simulink model "Case3_IEEE39_UGFLandGFM"  (R2024a)
settings: Solver=VariableStepAuto  StartTime=0.0  StopTime=30  RelTol=1e-3
InitFcn:
  | IEEE39data_UGFLandGFM;
values from neighbouring files (symbols this model uses):
  Fref = 60    [IEEE39data_UGFLandGFM.m]
  IBR = [ ... (first row only)    [IEEE39data_UGFLandGFM.m]
  line = [     1	2	0.0035	0.0411	0.6987	0	1	22 ... (first row only)    [IEEE39data_UGFLandGFM.m]
  Sbase = 1e6    (= 1000000)    [IEEE39data_UGFLandGFM.m]
  SG = [ ... (first row only)    [IEEE39data_UGFLandGFM.m]
  UGFML = [ ... (first row only)    [IEEE39data_UGFLandGFM.m]
  Vbase = 22e3    (= 22000)    [IEEE39data_UGFLandGFM.m]
libraries: spsThreePhaseVIMeasurementLib x66, spsThreePhasePISectionLineLib x35, spsPLL3phLib x25, spsControlledVoltageSourceLib x21, spsThreePhaseParallelRLCLoadLib x21, powerlib_extras x20, spsGroundLib x20, spsMeanLib x20, spsRMSLib x15, spsabctodq0Lib x11, spsThreePhaseSeriesRLCBranchLib x10, slpidlib x10
(part 2 of 5)

== system Case3_IEEE39_UGFLandGFM/SG1 ==
  3-phase Instantaneous Active & Reactive Power4 : powerlib_extras/Measurements/3-phase  Instantaneous  Active & Reactive Power
  Add : Sum  Inputs=+-
  Add1 : Sum  Inputs=-+
  Constant1 : Constant  Value=SG(1,6)
  Constant2 : Constant  Value=Fref
  Constant3 : Constant  Value=SG(1,4)
  Constant6 : Constant  Value=SG(1,7)
  Demux : Demux  Outputs=2
  Demux1 : Demux  Outputs=2
  Divide : Product  Inputs=*/
  Gain1 : Gain  Gain=0.2
  Gain2 : Gain  Gain=1.732/22000
  Mean : spsMeanLib/Mean  Freq=60  Vinit=0  Ts=1e-4
  PID Controller1 : slpidlib/PID Controller  Controller=PI  Form=Parallel  TimeDomain=Discrete-time  UseExternalTs=off  SampleTime=5e-4  IntegratorMethod=Forward Euler  FilterMethod=Forward Euler  ControllerParametersSource=internal  P=5  I=30  UseKiTs=off  D=0  UseExternalDerivativeSource=off  N=100  UseFilter=on  TunerSelectOption=Transfer Function Based (PID Tuner App)  InitialConditionSource=internal  InitialConditionForIntegrator=1  InitialConditionForFilter=0  DifferentiatorICPrevScaledInput=0  ExternalReset=level  TrackingMode=off  Kt=1  LimitOutput=off  SatLimitsSource=internal  UpperSaturationLimit=inf  LowerSaturationLimit=-inf  LinearizeAsGain=on  AntiWindupMode=none  Kb=1  LimitIntegrator=off  UpperIntegratorSaturationLimit=inf  LowerIntegratorSaturationLimit=-inf  POutMin=[]  POutMax=[]  IOutMin=[]  IOutMax=[]  DOutMin=[]  DOutMax=[]  NOutMin=[]  NOutMax=[]  SumOutMin=[]  SumOutMax=[]  SaturationOutMin=[]  SaturationOutMax=[]  PParamMin=[]  PParamMax=[]  IParamMin=[]  IParamMax=[]  DParamMin=[]  DParamMax=[]  NParamMin=[]  NParamMax=[]  KbParamMin=[]  KbParamMax=[]  KtParamMin=[]  KtParamMax=[]  KbOutMin=[]  KbOutMax=[]  KtOutMin=[]  KtOutMax=[]  IntegratorOutMin=[]  IntegratorOutMax=[]  FilterOutMin=[]  FilterOutMax=[]  SumI1OutMin=[]  SumI1OutMax=[]  SumI2OutMin=[]  SumI2OutMax=[]  SumI3OutMin=[]  SumI3OutMax=[]  SumI4OutMin=[]  SumI4OutMax=[]  SumDOutMin=[]  SumDOutMax=[]  DifferentiatorOutMin=[]  DifferentiatorOutMax=[]  FilterDiffOutCoefMin=[]  FilterDiffOutCoefMax=[]  ReciprocalOutMin=[]  ReciprocalOutMax=[]  SumDenOutMin=[]  SumDenOutMax=[]  SumNumOutMin=[]  SumNumOutMax=[]  DivideOutMin=[]  DivideOutMax=[]  UdiffTsProdOutMin=[]  UdiffTsProdOutMax=[]  NTsProdOutMin=[]  NTsProdOutMax=[]  UintegralTsProdOutMin=[]  UintegralTsProdOutMax=[]  UngainTsProdOutMin=[]  UngainTsProdOutMax=[]  ClampingZeroOutDataTypeStr=Inherit: Inherit via back propagation  ClampingZeroOutMin=[]  ClampingZeroOutMax=[]  FilterDenConstantOutDataTypeStr=Inherit: Inherit via back propagation  FilterDenConstantOutMin=[]  FilterDenConstantOutMax=[]  PCopyOutDataTypeStr=Inherit: Inherit via back propagation  PCopyOutMin=[]  PCopyOutMax=[]  NCopyOutDataTypeStr=Inherit: Inherit via back propagation  NCopyOutMin=[]  NCopyOutMax=[]  IntegratorContinuousStateAttributes=''  IntegratorStateMustResolveToSignalObject=off  IntegratorRTWStateStorageClass=Auto  FilterContinuousStateAttributes=''  FilterStateMustResolveToSignalObject=off  FilterRTWStateStorageClass=Auto  ParallelPVariant=InternalParameters  IdealPVariant=Disabled  IVariant=InternalParameters  DVariant=Disabled  IntegratorVariant=Discrete  SatVariant=Disabled  AWVariant=Passthrough  PCopyVariant=Disabled  TRVariant=Disabled  FdbkBlocksVariant=Forward  IdealPFdbkVariant=Disabled  SatFdbkVariant=Disabled  DerivativeFilterVariant=Disabled  NVariant=Disabled  NCopyVariant=Disabled_SignalSpec  FilterICVariant=Disabled  IntegratorICVariant=InternalICs  ExternalResetVariant=ExternalReset  TRSumVariant=Passthrough  SumFdbkVariant=Disabled  SumVariant=Sum_PI  TsampFilterVariant=InternalTs  TsampNgainVariant=Passthrough  TsampIntegralVariant=Disabled_SignalSpec  ExternalSaturationOutDataTypeStr=Inherit: Same as second input  DerivativeSourceVariant=Disabled
  PLL (3ph) : spsPLL3phLib/PLL (3ph)  Fmin=59.5  Par_Init=[0, 60]  ParK=[180, 3200, 1]  TcD=1e-4  MaxRateChangeFreq=12  FilterCutOffFreq=25  Ts=1e-5  AGC=on
  Product : Product
  RMS Measurement : eeRmsMeasurement/RMS Measurement  LabelModeActiveChoice=Total  F=60  SpecifyHarmonics=off  K=[0 1 2]  Ts=1e-4
      settings: LibrarySourceBlock=|
      | ee_sl_lib/Measurements/RMS
      | Measurement
  Saturation : Saturate  UpperLimit=1.2  LowerLimit=0.1
  Saturation2 : Saturate  UpperLimit=5  LowerLimit=0.5
  Scope : Scope  NumInputPorts=5
  Scope1 : Scope
  Step : Step  Before=1  After=0  SampleTime=0
  Sum : Sum  Inputs=|+-
  Synchronous Machine pu Standard : spsSynchronousMachinepuStandardLib/Synchronous Machine pu Standard  PresetModel=No  MechanicalLoad=Mechanical power Pm  ShowDetailedParameters=on  RotorType=Salient-pole  Units=per unit standard parameters  MeasurementBus=off  NominalParameters=[5e6 22000 60]  Reactances1=[ 1.81, 0.3, 0.23, 1.76, 0.65, 0.25, 0.15 ]  Reactances2=[2.24 0.17 0.12 1.02 0.13 0.08]  dAxisTimeConstants=Short-circuit  qAxisTimeConstants=Short-circuit  TimeConstants1="[ 4.4849  0.0681  0.1  ]"  TimeConstants2=[ 8.0, 0.03, 1.0, 0.07 ]  TimeConstants3="[  4.49  0.0681  0.0513  ]"  TimeConstants4=[ 8.0, 0.03, 0.3371, 0.0295 ]  TimeConstants5=[ 1.01, 0.053, 0.1 ]  TimeConstants6=[ 1.3201, 0.023, 1.0, 0.07 ]  TimeConstants7=[0.012 0.003 0.003]  TimeConstants8=[ 1.3201, 0.0231, 0.3371, 0.0295 ]  StatorResistance=0.037875  Mechanical=[SG(1,5) 0.02056 2]  PolePairs=20  InitialConditions="[ 0  0  0  0  0  0  0  0  1 ]"  SetSaturation=on  Saturation=[0.6404,0.7127,0.8441,0.9214,0.9956,1.082,1.19,1.316,1.457;0.7,0.7698,0.8872,0.9466,0.9969,1.046,1.1,1.151,1.201]  LoadFlowParameters=[1,0,0,0,0]  TsPowergui=0  TsBlock=-1  IterativeModel=Trapezoidal non iterative  IterativeDiscreteModel=Trapezoidal non iterative  BusType=PV  Pref=0  Qref=0  Qmin=-inf  Qmax=inf  PLF=0  QLF=0
  Three-Phase V-I Measurement3 : spsThreePhaseVIMeasurementLib/Three-Phase V-I Measurement  VoltageMeasurement=phase-to-ground  SetLabelV=off  LabelV=Vabc  Vpu=off  VpuLL=off  CurrentMeasurement=yes  SetLabelI=off  LabelI=Iabc  Ipu=off  Pbase=1e5  Vbase=380  OutputType=Complex  PhasorSimulation=off  PSBequivalent=0
  Transfer Fcn : TransferFcn  Denominator=[0.6 1]
  Conn1 : PMIOPort  Side=Right
  Conn2 : PMIOPort  Port=2  Side=Right
  Conn3 : PMIOPort  Port=3  Side=Right
  tag scope: P_Bus30=global, Q_Bus30=global, V_Bus30=global
  wires:
  3-phase Instantaneous Active & Reactive Power4/1 -> Mean/1
  Three-Phase V-I Measurement3/1 -> 3-phase Instantaneous Active & Reactive Power4/1, RMS Measurement/1, PLL (3ph)/1, Scope/1
  Three-Phase V-I Measurement3/2 -> Scope/2, 3-phase Instantaneous Active & Reactive Power4/2
  Mean/1 -> Demux1/1, Scope/3
  Add1/1 -> Gain1/1
  [SG_Freq] -> Add/1
  Constant2/1 -> Divide/2, Add/2
  Add/1 -> Divide/1
  Divide/1 -> Transfer Fcn/1
  Constant3/1 -> Product/2
  Constant1/1 -> Add1/2
  Product/1 -> Add1/1
  Transfer Fcn/1 -> Product/1
  Gain1/1 -> Saturation/1
  Gain2/1 -> Demux/1, Scope/4
  RMS Measurement/1 -> Gain2/1
  Demux/1 -> [V_Bus30], [VSG_pu]
  Constant6/1 -> Sum/1
  [VSG_pu] -> Sum/2
  PID Controller1/1 -> Saturation2/1
  Sum/1 -> PID Controller1/1
  Saturation/1 -> Synchronous Machine pu Standard/1
  PLL (3ph)/1 -> Scope/5, [SG_Freq]
  Demux1/1 -> [P_Bus30]
  Demux1/2 -> [Q_Bus30]
  Saturation2/1 -> Synchronous Machine pu Standard/2, Scope1/1
  Step/1 -> PID Controller1/2
  connections:
  Three-Phase V-I Measurement3/RConn1 -- Conn1/RConn1
  Three-Phase V-I Measurement3/RConn2 -- Conn2/RConn1
  Three-Phase V-I Measurement3/RConn3 -- Conn3/RConn1
  Three-Phase V-I Measurement3/LConn1 -- Synchronous Machine pu Standard/RConn1
  Three-Phase V-I Measurement3/LConn2 -- Synchronous Machine pu Standard/RConn2
  Three-Phase V-I Measurement3/LConn3 -- Synchronous Machine pu Standard/RConn3

== system Case3_IEEE39_UGFLandGFM/SG2 ==
  3-phase Instantaneous Active & Reactive Power4 : powerlib_extras/Measurements/3-phase  Instantaneous  Active & Reactive Power
  Add : Sum  Inputs=+-
  Add1 : Sum  Inputs=-+
  Constant1 : Constant  Value=SG(2,6)
  Constant2 : Constant  Value=Fref
  Constant3 : Constant  Value=SG(2,4)
  Constant5 : Constant  Commented=on  Value=1.1
  Constant6 : Constant  Value=SG(2,7)
  DC1A Excitation System : spsDC1AExcitationSystemLib/DC1A Excitation System  Commented=on  Tr=20e-3  KaTa=[460 0.006]  VRminmax=[-0.9 1.0]  KfTf=[0.05 1.5]  TbTc=[0 0]  KeTe=[0.05 0.46]  Efd12=[3.1 2.3]  SeEfd12=[0.33 0.10]  v0=[1 1.8]  TsBlock=0
      settings: LibrarySourceBlock=|
      | sps_lib/Electrical Machines/Synchronous Machine Control/DC1A
      | Excitation System
  Demux : Demux  Outputs=3
  Demux1 : Demux  Outputs=2
  Divide : Product  Inputs=*/
  From1 : From  Commented=on  GotoTag=VSG_pu
  Gain1 : Gain  Gain=0.2
  Gain2 : Gain  Gain=sqrt(3)/22000
  Ground : Ground  Commented=on
  Mean : spsMeanLib/Mean  Freq=60  Vinit=0  Ts=1e-4
  PID Controller1 : slpidlib/PID Controller  Controller=PI  Form=Parallel  TimeDomain=Discrete-time  UseExternalTs=off  SampleTime=5e-4  IntegratorMethod=Forward Euler  FilterMethod=Forward Euler  ControllerParametersSource=internal  P=5  I=30  UseKiTs=off  D=0  UseExternalDerivativeSource=off  N=100  UseFilter=on  TunerSelectOption=Transfer Function Based (PID Tuner App)  InitialConditionSource=internal  InitialConditionForIntegrator=1.8  InitialConditionForFilter=0  DifferentiatorICPrevScaledInput=0  ExternalReset=none  TrackingMode=off  Kt=1  LimitOutput=off  SatLimitsSource=internal  UpperSaturationLimit=inf  LowerSaturationLimit=-inf  LinearizeAsGain=on  AntiWindupMode=none  Kb=1  LimitIntegrator=off  UpperIntegratorSaturationLimit=inf  LowerIntegratorSaturationLimit=-inf  POutMin=[]  POutMax=[]  IOutMin=[]  IOutMax=[]  DOutMin=[]  DOutMax=[]  NOutMin=[]  NOutMax=[]  SumOutMin=[]  SumOutMax=[]  SaturationOutMin=[]  SaturationOutMax=[]  PParamMin=[]  PParamMax=[]  IParamMin=[]  IParamMax=[]  DParamMin=[]  DParamMax=[]  NParamMin=[]  NParamMax=[]  KbParamMin=[]  KbParamMax=[]  KtParamMin=[]  KtParamMax=[]  KbOutMin=[]  KbOutMax=[]  KtOutMin=[]  KtOutMax=[]  IntegratorOutMin=[]  IntegratorOutMax=[]  FilterOutMin=[]  FilterOutMax=[]  SumI1OutMin=[]  SumI1OutMax=[]  SumI2OutMin=[]  SumI2OutMax=[]  SumI3OutMin=[]  SumI3OutMax=[]  SumI4OutMin=[]  SumI4OutMax=[]  SumDOutMin=[]  SumDOutMax=[]  DifferentiatorOutMin=[]  DifferentiatorOutMax=[]  FilterDiffOutCoefMin=[]  FilterDiffOutCoefMax=[]  ReciprocalOutMin=[]  ReciprocalOutMax=[]  SumDenOutMin=[]  SumDenOutMax=[]  SumNumOutMin=[]  SumNumOutMax=[]  DivideOutMin=[]  DivideOutMax=[]  UdiffTsProdOutMin=[]  UdiffTsProdOutMax=[]  NTsProdOutMin=[]  NTsProdOutMax=[]  UintegralTsProdOutMin=[]  UintegralTsProdOutMax=[]  UngainTsProdOutMin=[]  UngainTsProdOutMax=[]  ClampingZeroOutDataTypeStr=Inherit: Inherit via back propagation  ClampingZeroOutMin=[]  ClampingZeroOutMax=[]  FilterDenConstantOutDataTypeStr=Inherit: Inherit via back propagation  FilterDenConstantOutMin=[]  FilterDenConstantOutMax=[]  PCopyOutDataTypeStr=Inherit: Inherit via back propagation  PCopyOutMin=[]  PCopyOutMax=[]  NCopyOutDataTypeStr=Inherit: Inherit via back propagation  NCopyOutMin=[]  NCopyOutMax=[]  IntegratorContinuousStateAttributes=''  IntegratorStateMustResolveToSignalObject=off  IntegratorRTWStateStorageClass=Auto  FilterContinuousStateAttributes=''  FilterStateMustResolveToSignalObject=off  FilterRTWStateStorageClass=Auto  ParallelPVariant=InternalParameters  IdealPVariant=Disabled  IVariant=InternalParameters  DVariant=Disabled  IntegratorVariant=Discrete  SatVariant=Disabled  AWVariant=Passthrough  PCopyVariant=Disabled  TRVariant=Disabled  FdbkBlocksVariant=Forward  IdealPFdbkVariant=Disabled  SatFdbkVariant=Disabled  DerivativeFilterVariant=Disabled  NVariant=Disabled  NCopyVariant=Disabled_SignalSpec  FilterICVariant=Disabled  IntegratorICVariant=InternalICs  ExternalResetVariant=Disabled  TRSumVariant=Passthrough  SumFdbkVariant=Disabled  SumVariant=Sum_PI  TsampFilterVariant=InternalTs  TsampNgainVariant=Passthrough  TsampIntegralVariant=Disabled_SignalSpec  ExternalSaturationOutDataTypeStr=Inherit: Same as second input  DerivativeSourceVariant=Disabled
  PLL (3ph) : spsPLL3phLib/PLL (3ph)  Fmin=59.5  Par_Init=[0, 60]  ParK=[180, 3200, 1]  TcD=1e-4  MaxRateChangeFreq=12  FilterCutOffFreq=25  Ts=1e-5  AGC=on
  Product : Product
  RMS Measurement : eeRmsMeasurement/RMS Measurement  LabelModeActiveChoice=Total  F=60  SpecifyHarmonics=off  K=[0 1 2]  Ts=1e-4
      settings: LibrarySourceBlock=|
      | ee_sl_lib/Measurements/RMS
      | Measurement
  Saturation : Saturate  UpperLimit=0.9  LowerLimit=0.1
  Saturation1 : Saturate  Commented=on  UpperLimit=4  LowerLimit=1.5
  Saturation2 : Saturate  UpperLimit=5  LowerLimit=0.9
  Scope : Scope  NumInputPorts=5
  Scope{1..4} (4 alike) : Scope
  Sum : Sum  Inputs=|+-
  Synchronous Machine pu Standard : spsSynchronousMachinepuStandardLib/Synchronous Machine pu Standard  PresetModel=No  MechanicalLoad=Mechanical power Pm  ShowDetailedParameters=on  RotorType=Salient-pole  Units=per unit standard parameters  MeasurementBus=off  NominalParameters=[5e6 22000 60]  Reactances1=[ 1.81, 0.3, 0.23, 1.76, 0.65, 0.25, 0.15 ]  Reactances2=[2.24 0.17 0.12 1.02 0.13 0.08]  dAxisTimeConstants=Short-circuit  qAxisTimeConstants=Short-circuit  TimeConstants1="[ 4.4849  0.0681  0.1  ]"  TimeConstants2=[ 8.0, 0.03, 1.0, 0.07 ]  TimeConstants3="[  4.49  0.0681  0.0513  ]"  TimeConstants4=[ 8.0, 0.03, 0.3371, 0.0295 ]  TimeConstants5=[ 1.01, 0.053, 0.1 ]  TimeConstants6=[ 1.3201, 0.023, 1.0, 0.07 ]  TimeConstants7=[0.012 0.003 0.003]  TimeConstants8=[ 1.3201, 0.0231, 0.3371, 0.0295 ]  StatorResistance=0.037875  Mechanical=[SG(2,5) 0.02056 2]  PolePairs=20  InitialConditions="[ 0  0  0  0  0  0  0  0  1 ]"  SetSaturation=on  Saturation=[0.6404,0.7127,0.8441,0.9214,0.9956,1.082,1.19,1.316,1.457;0.7,0.7698,0.8872,0.9466,0.9969,1.046,1.1,1.151,1.201]  LoadFlowParameters=[1,0,0,0,0]  TsPowergui=0  TsBlock=-1  IterativeModel=Trapezoidal non iterative  IterativeDiscreteModel=Trapezoidal non iterative  BusType=PV  Pref=0  Qref=0  Qmin=-inf  Qmax=inf  PLF=0  QLF=0
  Three-Phase V-I Measurement3 : spsThreePhaseVIMeasurementLib/Three-Phase V-I Measurement  VoltageMeasurement=phase-to-ground  SetLabelV=off  LabelV=Vabc  Vpu=off  VpuLL=off  CurrentMeasurement=yes  SetLabelI=off  LabelI=Iabc  Ipu=off  Pbase=1e5  Vbase=380  OutputType=Complex  PhasorSimulation=off  PSBequivalent=0
  Transfer Fcn : TransferFcn  Denominator=[0.6 1]
  Conn1 : PMIOPort  Side=Right
  Conn2 : PMIOPort  Port=2  Side=Right
  Conn3 : PMIOPort  Port=3  Side=Right
  tag scope: P_Bus33=global, Q_Bus33=global, V_Bus33=global
  wires:
  3-phase Instantaneous Active & Reactive Power4/1 -> Mean/1
  Three-Phase V-I Measurement3/1 -> 3-phase Instantaneous Active & Reactive Power4/1, RMS Measurement/1, PLL (3ph)/1, Scope/1
  Three-Phase V-I Measurement3/2 -> Scope/2, 3-phase Instantaneous Active & Reactive Power4/2
  Mean/1 -> Demux1/1, Scope/3
  Add1/1 -> Gain1/1
  [SG_Freq] -> Add/1
  Constant2/1 -> Divide/2, Add/2
  Add/1 -> Divide/1
  Divide/1 -> [deltaw_SG], Transfer Fcn/1
  Constant3/1 -> Product/2
  Constant1/1 -> Add1/2
  Product/1 -> Add1/1
  Transfer Fcn/1 -> Product/1
  Gain1/1 -> Saturation/1
  Gain2/1 -> Demux/1, Scope/4
  RMS Measurement/1 -> Gain2/1
  From1/1 -> DC1A Excitation System/2
  Constant5/1 -> DC1A Excitation System/1
  Ground/1 -> DC1A Excitation System/3
  Demux/1 -> [V_Bus33], [VSG_pu]
  DC1A Excitation System/1 -> Saturation1/1
  Constant6/1 -> Sum/1
  [VSG_pu] -> Sum/2
  PID Controller1/1 -> Saturation2/1
  Sum/1 -> Scope4/1, PID Controller1/1
  Saturation/1 -> Synchronous Machine pu Standard/1
  PLL (3ph)/1 -> Scope/5, [SG_Freq]
  Saturation2/1 -> Scope1/1, Synchronous Machine pu Standard/2, Scope3/1, Scope2/1
  Demux1/1 -> [P_Bus33]
  Demux1/2 -> [Q_Bus33]
  connections:
  Three-Phase V-I Measurement3/RConn1 -- Conn1/RConn1
  Three-Phase V-I Measurement3/RConn2 -- Conn2/RConn1
  Three-Phase V-I Measurement3/RConn3 -- Conn3/RConn1
  Three-Phase V-I Measurement3/LConn1 -- Synchronous Machine pu Standard/RConn1
  Three-Phase V-I Measurement3/LConn2 -- Synchronous Machine pu Standard/RConn2
  Three-Phase V-I Measurement3/LConn3 -- Synchronous Machine pu Standard/RConn3

== system Case3_IEEE39_UGFLandGFM/SG3 ==
  3-phase Instantaneous Active & Reactive Power4 : powerlib_extras/Measurements/3-phase  Instantaneous  Active & Reactive Power
  Add : Sum  Inputs=+-
  Add1 : Sum  Inputs=-+
  Constant1 : Constant  Value=SG(3,6)
  Constant2 : Constant  Value=Fref
  Constant3 : Constant  Value=SG(3,4)
  Constant6 : Constant  Value=SG(3,7)
  Demux : Demux  Outputs=2
  Demux1 : Demux  Outputs=2
  Divide : Product  Inputs=*/
  Gain1 : Gain  Gain=0.2
  Gain2 : Gain  Gain=1.732/22000
  Mean : spsMeanLib/Mean  Freq=60  Vinit=0  Ts=1e-4
  PID Controller1 : slpidlib/PID Controller  Controller=PI  Form=Parallel  TimeDomain=Discrete-time  UseExternalTs=off  SampleTime=5e-4  IntegratorMethod=Forward Euler  FilterMethod=Forward Euler  ControllerParametersSource=internal  P=5  I=30  UseKiTs=off  D=0  UseExternalDerivativeSource=off  N=100  UseFilter=on  TunerSelectOption=Transfer Function Based (PID Tuner App)  InitialConditionSource=internal  InitialConditionForIntegrator=1.8  InitialConditionForFilter=0  DifferentiatorICPrevScaledInput=0  ExternalReset=none  TrackingMode=off  Kt=1  LimitOutput=off  SatLimitsSource=internal  UpperSaturationLimit=inf  LowerSaturationLimit=-inf  LinearizeAsGain=on  AntiWindupMode=none  Kb=1  LimitIntegrator=off  UpperIntegratorSaturationLimit=inf  LowerIntegratorSaturationLimit=-inf  POutMin=[]  POutMax=[]  IOutMin=[]  IOutMax=[]  DOutMin=[]  DOutMax=[]  NOutMin=[]  NOutMax=[]  SumOutMin=[]  SumOutMax=[]  SaturationOutMin=[]  SaturationOutMax=[]  PParamMin=[]  PParamMax=[]  IParamMin=[]  IParamMax=[]  DParamMin=[]  DParamMax=[]  NParamMin=[]  NParamMax=[]  KbParamMin=[]  KbParamMax=[]  KtParamMin=[]  KtParamMax=[]  KbOutMin=[]  KbOutMax=[]  KtOutMin=[]  KtOutMax=[]  IntegratorOutMin=[]  IntegratorOutMax=[]  FilterOutMin=[]  FilterOutMax=[]  SumI1OutMin=[]  SumI1OutMax=[]  SumI2OutMin=[]  SumI2OutMax=[]  SumI3OutMin=[]  SumI3OutMax=[]  SumI4OutMin=[]  SumI4OutMax=[]  SumDOutMin=[]  SumDOutMax=[]  DifferentiatorOutMin=[]  DifferentiatorOutMax=[]  FilterDiffOutCoefMin=[]  FilterDiffOutCoefMax=[]  ReciprocalOutMin=[]  ReciprocalOutMax=[]  SumDenOutMin=[]  SumDenOutMax=[]  SumNumOutMin=[]  SumNumOutMax=[]  DivideOutMin=[]  DivideOutMax=[]  UdiffTsProdOutMin=[]  UdiffTsProdOutMax=[]  NTsProdOutMin=[]  NTsProdOutMax=[]  UintegralTsProdOutMin=[]  UintegralTsProdOutMax=[]  UngainTsProdOutMin=[]  UngainTsProdOutMax=[]  ClampingZeroOutDataTypeStr=Inherit: Inherit via back propagation  ClampingZeroOutMin=[]  ClampingZeroOutMax=[]  FilterDenConstantOutDataTypeStr=Inherit: Inherit via back propagation  FilterDenConstantOutMin=[]  FilterDenConstantOutMax=[]  PCopyOutDataTypeStr=Inherit: Inherit via back propagation  PCopyOutMin=[]  PCopyOutMax=[]  NCopyOutDataTypeStr=Inherit: Inherit via back propagation  NCopyOutMin=[]  NCopyOutMax=[]  IntegratorContinuousStateAttributes=''  IntegratorStateMustResolveToSignalObject=off  IntegratorRTWStateStorageClass=Auto  FilterContinuousStateAttributes=''  FilterStateMustResolveToSignalObject=off  FilterRTWStateStorageClass=Auto  ParallelPVariant=InternalParameters  IdealPVariant=Disabled  IVariant=InternalParameters  DVariant=Disabled  IntegratorVariant=Discrete  SatVariant=Disabled  AWVariant=Passthrough  PCopyVariant=Disabled  TRVariant=Disabled  FdbkBlocksVariant=Forward  IdealPFdbkVariant=Disabled  SatFdbkVariant=Disabled  DerivativeFilterVariant=Disabled  NVariant=Disabled  NCopyVariant=Disabled_SignalSpec  FilterICVariant=Disabled  IntegratorICVariant=InternalICs  ExternalResetVariant=Disabled  TRSumVariant=Passthrough  SumFdbkVariant=Disabled  SumVariant=Sum_PI  TsampFilterVariant=InternalTs  TsampNgainVariant=Passthrough  TsampIntegralVariant=Disabled_SignalSpec  ExternalSaturationOutDataTypeStr=Inherit: Same as second input  DerivativeSourceVariant=Disabled
  PLL (3ph) : spsPLL3phLib/PLL (3ph)  Fmin=59.5  Par_Init=[0, 60]  ParK=[180, 3200, 1]  TcD=1e-4  MaxRateChangeFreq=12  FilterCutOffFreq=25  Ts=1e-5  AGC=on
  Product : Product
  RMS Measurement : eeRmsMeasurement/RMS Measurement  LabelModeActiveChoice=Total  F=60  SpecifyHarmonics=off  K=[0 1 2]  Ts=1e-4
      settings: LibrarySourceBlock=|
      | ee_sl_lib/Measurements/RMS
      | Measurement
  Saturation : Saturate  UpperLimit=0.9  LowerLimit=0.1
  Saturation2 : Saturate  UpperLimit=5  LowerLimit=0.9
  Scope : Scope  NumInputPorts=5
  Sum : Sum  Inputs=|+-
  Synchronous Machine pu Standard : spsSynchronousMachinepuStandardLib/Synchronous Machine pu Standard  PresetModel=No  MechanicalLoad=Mechanical power Pm  ShowDetailedParameters=on  RotorType=Salient-pole  Units=per unit standard parameters  MeasurementBus=off  NominalParameters=[5e6 22000 60]  Reactances1=[ 1.81, 0.3, 0.23, 1.76, 0.65, 0.25, 0.15 ]  Reactances2=[2.24 0.17 0.12 1.02 0.13 0.08]  dAxisTimeConstants=Short-circuit  qAxisTimeConstants=Short-circuit  TimeConstants1="[ 4.4849  0.0681  0.1  ]"  TimeConstants2=[ 8.0, 0.03, 1.0, 0.07 ]  TimeConstants3="[  4.49  0.0681  0.0513  ]"  TimeConstants4=[ 8.0, 0.03, 0.3371, 0.0295 ]  TimeConstants5=[ 1.01, 0.053, 0.1 ]  TimeConstants6=[ 1.3201, 0.023, 1.0, 0.07 ]  TimeConstants7=[0.012 0.003 0.003]  TimeConstants8=[ 1.3201, 0.0231, 0.3371, 0.0295 ]  StatorResistance=0.037875  Mechanical=[SG(3,5) 0.02056 2]  PolePairs=20  InitialConditions="[ 0  0  0  0  0  0  0  0  1 ]"  SetSaturation=on  Saturation=[0.6404,0.7127,0.8441,0.9214,0.9956,1.082,1.19,1.316,1.457;0.7,0.7698,0.8872,0.9466,0.9969,1.046,1.1,1.151,1.201]  LoadFlowParameters=[1,0,0,0,0]  TsPowergui=0  TsBlock=-1  IterativeModel=Trapezoidal non iterative  IterativeDiscreteModel=Trapezoidal non iterative  BusType=PV  Pref=0  Qref=0  Qmin=-inf  Qmax=inf  PLF=0  QLF=0
  Three-Phase V-I Measurement3 : spsThreePhaseVIMeasurementLib/Three-Phase V-I Measurement  VoltageMeasurement=phase-to-ground  SetLabelV=off  LabelV=Vabc  Vpu=off  VpuLL=off  CurrentMeasurement=yes  SetLabelI=off  LabelI=Iabc  Ipu=off  Pbase=1e5  Vbase=380  OutputType=Complex  PhasorSimulation=off  PSBequivalent=0
  Transfer Fcn : TransferFcn  Denominator=[0.6 1]
  Conn1 : PMIOPort  Side=Right
  Conn2 : PMIOPort  Port=2  Side=Right
  Conn3 : PMIOPort  Port=3  Side=Right
  tag scope: P_Bus34=global, Q_Bus34=global, V_Bus34=global
  wires:
  3-phase Instantaneous Active & Reactive Power4/1 -> Mean/1
  Three-Phase V-I Measurement3/1 -> 3-phase Instantaneous Active & Reactive Power4/1, RMS Measurement/1, PLL (3ph)/1, Scope/1
  Three-Phase V-I Measurement3/2 -> Scope/2, 3-phase Instantaneous Active & Reactive Power4/2
  Mean/1 -> Demux1/1, Scope/3
  Add1/1 -> Gain1/1
  Saturation2/1 -> Synchronous Machine pu Standard/2
  [SG_Freq] -> Add/1
  Constant2/1 -> Divide/2, Add/2
  Add/1 -> Divide/1
  Divide/1 -> [deltaw_SG], Transfer Fcn/1
  Constant3/1 -> Product/2
  Constant1/1 -> Add1/2
  Product/1 -> Add1/1
  Transfer Fcn/1 -> Product/1
  Gain1/1 -> Saturation/1
  Gain2/1 -> Demux/1, Scope/4
  RMS Measurement/1 -> Gain2/1
  Demux/1 -> [V_Bus34], [VSG_pu]
  Constant6/1 -> Sum/1
  [VSG_pu] -> Sum/2
  PID Controller1/1 -> Saturation2/1
  Sum/1 -> PID Controller1/1
  Saturation/1 -> Synchronous Machine pu Standard/1
  PLL (3ph)/1 -> Scope/5, [SG_Freq]
  Demux1/1 -> [P_Bus34]
  Demux1/2 -> [Q_Bus34]
  connections:
  Three-Phase V-I Measurement3/RConn1 -- Conn1/RConn1
  Three-Phase V-I Measurement3/RConn2 -- Conn2/RConn1
  Three-Phase V-I Measurement3/RConn3 -- Conn3/RConn1
  Three-Phase V-I Measurement3/LConn1 -- Synchronous Machine pu Standard/RConn1
  Three-Phase V-I Measurement3/LConn2 -- Synchronous Machine pu Standard/RConn2
  Three-Phase V-I Measurement3/LConn3 -- Synchronous Machine pu Standard/RConn3

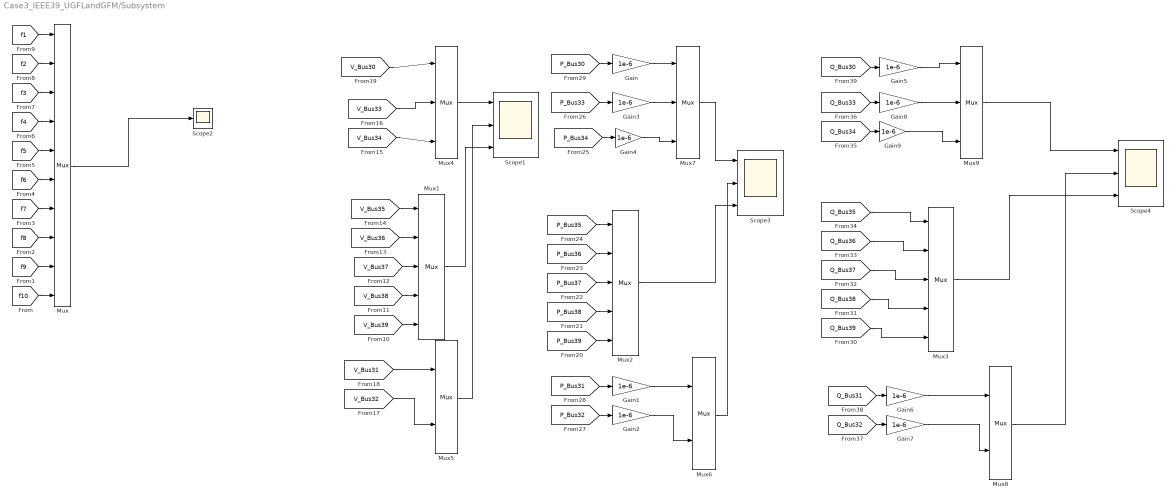
== system Case3_IEEE39_UGFLandGFM/Subsystem ==
  Gain{,1..9} (10 alike) : Gain  Gain=1e-6
  Mux : Mux  Inputs=10
  Mux1 : Mux  Inputs=5
  Mux2 : Mux  Inputs=5
  Mux3 : Mux  Inputs=5
  Mux4 : Mux  Inputs=3
  Mux5 : Mux  Inputs=2
  Mux6 : Mux  Inputs=2
  Mux7 : Mux  Inputs=3
  Mux8 : Mux  Inputs=2
  Mux9 : Mux  Inputs=3
  Scope1 : Scope  NumInputPorts=3
  Scope2 : Scope
  Scope3 : Scope  NumInputPorts=3
  Scope4 : Scope  NumInputPorts=3
  wires:
  [f10] -> Mux/10
  [f1] -> Mux/1
  [f2] -> Mux/2
  [f3] -> Mux/3
  [f4] -> Mux/4
  [f5] -> Mux/5
  [f6] -> Mux/6
  [f7] -> Mux/7
  [f8] -> Mux/8
  [f9] -> Mux/9
  Mux/1 -> Scope2/1
  [V_Bus36] -> Mux1/2
  [V_Bus38] -> Mux1/4
  [V_Bus34] -> Mux4/3
  [V_Bus30] -> Mux4/1
  [V_Bus37] -> Mux1/3
  Mux4/1 -> Scope1/1
  [V_Bus33] -> Mux4/2
  [V_Bus35] -> Mux1/1
  [V_Bus32] -> Mux5/2
  [V_Bus39] -> Mux1/5
  [V_Bus31] -> Mux5/1
  [P_Bus30] -> Gain/1
  [P_Bus37] -> Mux2/3
  [P_Bus36] -> Mux2/2
  [P_Bus35] -> Mux2/1
  [P_Bus38] -> Mux2/4
  Mux2/1 -> Scope3/3
  [P_Bus39] -> Mux2/5
  [P_Bus31] -> Gain1/1
  [Q_Bus38] -> Mux3/4
  [Q_Bus39] -> Mux3/5
  [Q_Bus37] -> Mux3/3
  [Q_Bus36] -> Mux3/2
  [Q_Bus35] -> Mux3/1
  [P_Bus32] -> Gain2/1
  [P_Bus33] -> Gain3/1
  [P_Bus34] -> Gain4/1
  [Q_Bus30] -> Gain5/1
  [Q_Bus31] -> Gain6/1
  [Q_Bus32] -> Gain7/1
  [Q_Bus33] -> Gain8/1
  [Q_Bus34] -> Gain9/1
  Mux1/1 -> Scope1/3
  Mux5/1 -> Scope1/2
  Gain1/1 -> Mux6/1
  Gain2/1 -> Mux6/2
  Mux6/1 -> Scope3/2
  Gain/1 -> Mux7/1
  Gain3/1 -> Mux7/2
  Gain4/1 -> Mux7/3
  Gain6/1 -> Mux8/1
  Gain7/1 -> Mux8/2
  Mux9/1 -> Scope4/1
  Gain8/1 -> Mux9/2
  Gain5/1 -> Mux9/1
  Gain9/1 -> Mux9/3
  Mux7/1 -> Scope3/1
  Mux8/1 -> Scope4/2
  Mux3/1 -> Scope4/3

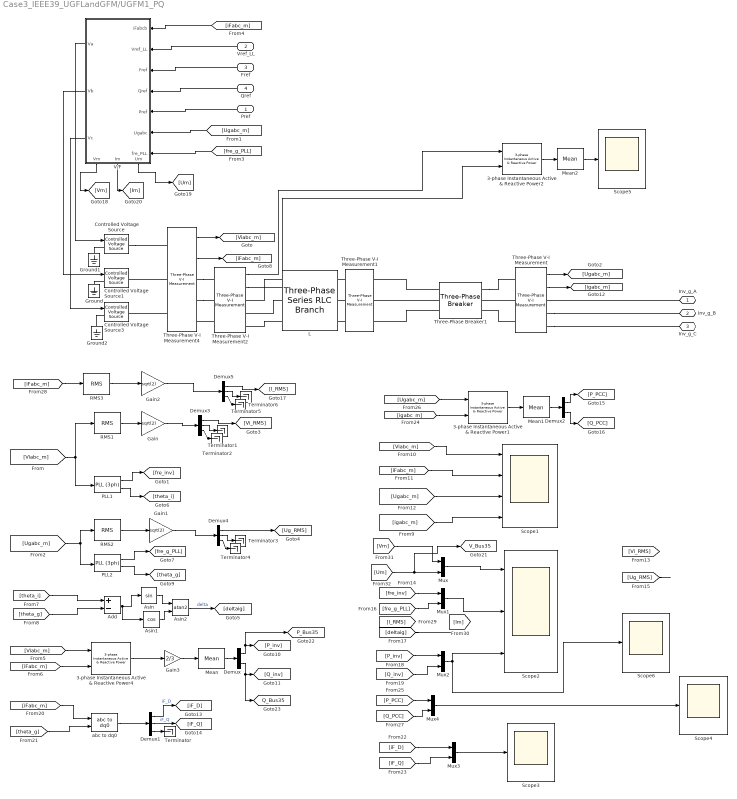
== system Case3_IEEE39_UGFLandGFM/UGFM1_PQ ==
  Pref : Inport
  Vref_LL : Inport  Port=2
  Fref : Inport  Port=3
  Qref : Inport  Port=4
  3-phase Instantaneous Active & Reactive Power1 : powerlib_extras/Measurements/3-phase  Instantaneous  Active & Reactive Power
  3-phase Instantaneous Active & Reactive Power2 : powerlib_extras/Measurements/3-phase  Instantaneous  Active & Reactive Power
  3-phase Instantaneous Active & Reactive Power4 : powerlib_extras/Measurements/3-phase  Instantaneous  Active & Reactive Power
  Add : Sum  Inputs=+-
  Asin : Trigonometry
  Asin1 : Trigonometry  Operator=cos
  Asin2 : Trigonometry  Operator=atan2
  Controlled Voltage Source : spsControlledVoltageSourceLib/Controlled Voltage Source  Initialize=on  Source_Type=DC  Amplitude=300  Phase=0  Frequency=60  Measurements=None
  Controlled Voltage Source1 : spsControlledVoltageSourceLib/Controlled Voltage Source  Initialize=on  Source_Type=DC  Amplitude=300  Phase=-120  Frequency=60  Measurements=None
  Controlled Voltage Source3 : spsControlledVoltageSourceLib/Controlled Voltage Source  Initialize=on  Source_Type=DC  Amplitude=300  Phase=120  Frequency=60  Measurements=None
  Demux : Demux  Outputs=2
  Demux{1,3..5} (4 alike) : Demux  Outputs=3
  Demux2 : Demux  Outputs=2
  Gain : Gain  Gain=sqrt(2)
  Gain1 : Gain  Gain=sqrt(2)
  Gain2 : Gain  Gain=sqrt(2)
  Gain3 : Gain  Gain=2/3
  Ground : spsGroundLib/Ground  LConnTagsString=a
  Ground1 : spsGroundLib/Ground  LConnTagsString=a
  Ground2 : spsGroundLib/Ground  LConnTagsString=a
  L : spsThreePhaseSeriesRLCBranchLib/Three-Phase Series RLC Branch  LConnTagsString=A|B|C  RConnTagsString=A|B|C  BranchType=RL  Resistance=0.05*Vbase^2/Sbase  Inductance=0.05*(Vbase^2/Sbase/377)  Capacitance=1.0  Measurements=None
  Mean : spsMeanLib/Mean  Freq=60  Vinit=0  Ts=5e-4
  Mean1 : spsMeanLib/Mean  Freq=60  Vinit=0  Ts=1e-4
  Mean2 : spsMeanLib/Mean  Freq=60  Vinit=0  Ts=5e-4
  Mux{,1..4} (5 alike) : Mux  Inputs=2
  PLL1 : spsPLL3phLib/PLL (3ph)  Fmin=35  Par_Init=[0, 60]  ParK=[180, 3200, 1]  TcD=1e-4  MaxRateChangeFreq=12  FilterCutOffFreq=25  Ts=1e-5  AGC=on
  PLL2 : spsPLL3phLib/PLL (3ph)  Fmin=35  Par_Init=[0, 60]  ParK=[180, 3200, 1]  TcD=1e-4  MaxRateChangeFreq=12  FilterCutOffFreq=25  Ts=1e-5  AGC=on
  RMS1 : spsRMSLib/RMS  TrueRMS=on  Freq=60  RMSInit=1  Ts=1e-4
  RMS2 : spsRMSLib/RMS  TrueRMS=on  Freq=60  RMSInit=1  Ts=1e-4
  RMS3 : spsRMSLib/RMS  TrueRMS=on  Freq=60  RMSInit=1  Ts=5e-4
  Scope1 : Scope  NumInputPorts=4
  Scope2 : Scope  NumInputPorts=3
  Scope{3..6} (4 alike) : Scope
  Terminator{,1..6} (7 alike) : Terminator
  Three-Phase V-I Measurement : spsThreePhaseVIMeasurementLib/Three-Phase V-I Measurement  VoltageMeasurement=phase-to-ground  SetLabelV=off  LabelV=Vabc  Vpu=on  VpuLL=off  CurrentMeasurement=yes  SetLabelI=off  LabelI=Iabc  Ipu=on  Pbase=Sbase  Vbase=Vbase  OutputType=Complex  PhasorSimulation=off  PSBequivalent=0
  Three-Phase V-I Measurement1 : spsThreePhaseVIMeasurementLib/Three-Phase V-I Measurement  VoltageMeasurement=no  SetLabelV=off  LabelV=Vabc  Vpu=off  VpuLL=off  CurrentMeasurement=no  SetLabelI=off  LabelI=Iabc  Ipu=off  Pbase=1e5  Vbase=380  OutputType=Complex  PhasorSimulation=off  PSBequivalent=0
  Three-Phase V-I Measurement2 : spsThreePhaseVIMeasurementLib/Three-Phase V-I Measurement  VoltageMeasurement=phase-to-ground  SetLabelV=off  LabelV=Vabc  Vpu=off  VpuLL=off  CurrentMeasurement=yes  SetLabelI=off  LabelI=Iabc  Ipu=off  Pbase=Sbase  Vbase=Vbase  OutputType=Complex  PhasorSimulation=off  PSBequivalent=0
  Three-Phase V-I Measurement4 : spsThreePhaseVIMeasurementLib/Three-Phase V-I Measurement  VoltageMeasurement=phase-to-ground  SetLabelV=off  LabelV=u  Vpu=on  VpuLL=off  CurrentMeasurement=yes  SetLabelI=off  LabelI=iFabcp3  Ipu=on  Pbase=Sbase  Vbase=Vbase  OutputType=Complex  PhasorSimulation=off  PSBequivalent=0
  Three-Phase Breaker1 : spsThreePhaseBreakerLib/Three-Phase Breaker  InitialState=open  SwitchA=on  SwitchB=on  SwitchC=on  SwitchTimes=[0.1]  External=off  BreakerResistance=0.0001  SnubberResistance=1e8  SnubberCapacitance=inf  Measurements=None
  V/F : Subsystem
      settings: PortSchema="{\"entries\":[{\"content\":{\"sides\":[{\"content\":{\"connectorIds\":[\"In1\",\"In2\",\"In3\",\"In4\",\"In5\",\"In6\",\"In7\"]},\"type\":\"ConnectorPlacement.EquallySpacedRectSide\",\"uuid\":\"ccc7dc11-36db-4369-953c-0655fd1e2442\"},{\"content\":{\"connectorIds\":[\"Out1\",\"Out2\",\"Out3\"],\"side\":\"RIGHT\"},\"type\":\"ConnectorPlacement.EquallySpacedRectSide\",\"uuid\":\"5735cf9b-d8e4-4bce-b2db-12738d0d9e4d\"},{\"content\":{\"side\":\"TOP\"},\"type\":\"ConnectorPlacement.EquallySpacedRectSide\",\"uuid\":\"e010782d-2644-4ebf-978f-8395ad947d0e\"},{\"content\":{\"connectorIds\":[\"Out4\",\"Out5\",\"Out6\"],\"side\":\"BOTTOM\"},\"type\":\"ConnectorPlacement.EquallySpacedRectSide\",\"uuid\":\"5965ef6f-6121-4d63-9a5a-1f7a3d153058\"}]},\"type\":\"ConnectorPlacement.EquallySpacedConnector\",\"uuid\":\"be33ea6e-20ef-4fc3-81eb-341d11cc9c18\"}],\"packageUris\":[\"http://schema.mathworks.com/mf0/Connector/R2020b\"],\"version\":\"1.0\"}"
  abc to dq0 : spsabctodq0Lib/abc to dq0  Alignment=90 degrees behind phase A axis
  Inv_g_A : PMIOPort  Side=Right
  Inv_g_B : PMIOPort  Port=2  Side=Right
  Inv_g_C : PMIOPort  Port=3  Side=Right
  tag scope: P_Bus35=global, Q_Bus35=global, V_Bus35=global
  wires:
  Three-Phase V-I Measurement/1 -> [Ugabc_m]
  Vref_LL/1 -> V/F/2(Vref_LL)
  V/F/2(Vb) -> Controlled Voltage Source1/1
  V/F/3(Vc) -> Controlled Voltage Source3/1
  Pref/1 -> V/F/5(Pref)
  Qref/1 -> V/F/4(Qref)
  Fref/1 -> V/F/3(Fref)
  RMS1/1 -> Gain/1
  Three-Phase V-I Measurement4/1 -> [Viabc_m]
  [Viabc_m] -> RMS1/1, PLL1/1
  PLL1/2 -> [theta_i]
  PLL1/1 -> [fre_inv]
  [Ugabc_m] -> V/F/6(Ugabc)
  [Ugabc_m] -> PLL2/1, RMS2/1
  RMS2/1 -> Gain1/1
  PLL2/2 -> [theta_g]
  PLL2/1 -> [fre_g_PLL]
  Three-Phase V-I Measurement4/2 -> [iFabc_m]
  [iFabc_m] -> V/F/1(iFabcb)
  [Viabc_m] -> 3-phase Instantaneous Active & Reactive Power4/1
  [iFabc_m] -> 3-phase Instantaneous Active & Reactive Power4/2
  Mean/1 -> Demux/1
  Demux/1 -> [P_Bus35], [P_inv]
  Demux/2 -> [Q_Bus35], [Q_inv]
  Three-Phase V-I Measurement/2 -> [igabc_m]
  [Viabc_m] -> Scope1/1
  [iFabc_m] -> Scope1/2
  [Ugabc_m] -> Scope1/3
  [igabc_m] -> Scope1/4
  [fre_inv] -> Mux1/1
  [Ug_RMS] -> ?
  Mux/1 -> Scope2/1
  [fre_g_PLL] -> Mux1/2
  Mux1/1 -> Scope2/2
  [deltaig] -> ?
  [P_inv] -> Mux2/1
  [Q_inv] -> Mux2/2
  Mux2/1 -> Scope2/3, Scope6/1
  Gain/1 -> Demux3/1
  [fre_g_PLL] -> V/F/7(fre_PLL)
  [theta_i] -> Add/1
  Add/1 -> Asin/1, Asin1/1
  [theta_g] -> Add/2
  Asin/1 -> Asin2/1
  Asin1/1 -> Asin2/2
  Asin2/1 -> [deltaig]  "delta"
  [iFabc_m] -> abc to dq0/1
  [theta_g] -> abc to dq0/2
  abc to dq0/1 -> Demux1/1
  Demux1/3 -> Terminator/1
  Demux1/1 -> [iF_D]  "iF_D"
  Demux1/2 -> [iF_Q]  "iF_Q"
  [iF_D] -> Mux3/1
  [iF_Q] -> Mux3/2
  Mux3/1 -> Scope3/1
  V/F/1(Va) -> Controlled Voltage Source/1
  Demux2/2 -> [Q_PCC]
  [Ugabc_m] -> 3-phase Instantaneous Active & Reactive Power1/1
  [igabc_m] -> 3-phase Instantaneous Active & Reactive Power1/2
  Mean1/1 -> Demux2/1
  Demux2/1 -> [P_PCC]
  3-phase Instantaneous Active & Reactive Power1/1 -> Mean1/1
  [P_PCC] -> Mux4/1
  [Q_PCC] -> Mux4/2
  Mux4/1 -> Scope4/1
  Demux3/1 -> [Vi_RMS]
  Demux3/2 -> Terminator1/1
  Demux3/3 -> Terminator2/1
  Demux4/3 -> Terminator4/1
  Demux4/1 -> [Ug_RMS]
  Demux4/2 -> Terminator3/1
  Gain1/1 -> Demux4/1
  [iFabc_m] -> RMS3/1
  RMS3/1 -> Gain2/1
  Demux5/3 -> Terminator6/1
  Demux5/1 -> [I_RMS]
  Demux5/2 -> Terminator5/1
  Gain2/1 -> Demux5/1
  Three-Phase V-I Measurement2/1 -> 3-phase Instantaneous Active & Reactive Power2/1
  Mean2/1 -> Scope5/1
  Three-Phase V-I Measurement2/2 -> 3-phase Instantaneous Active & Reactive Power2/2
  3-phase Instantaneous Active & Reactive Power2/1 -> Mean2/1
  Gain3/1 -> Mean/1
  3-phase Instantaneous Active & Reactive Power4/1 -> Gain3/1
  [Vm] -> Mux/1
  [Um] -> [V_Bus35], Mux/2
  V/F/5(Im) -> [Im]
  V/F/6(Vm) -> [Vm]
  V/F/4(Um) -> [Um]
  connections:
  Three-Phase V-I Measurement/RConn2 -- Inv_g_B/RConn1
  Three-Phase V-I Measurement4/LConn2 -- Controlled Voltage Source1/RConn1
  Controlled Voltage Source/RConn1 -- Three-Phase V-I Measurement4/LConn1
  Three-Phase V-I Measurement4/LConn3 -- Controlled Voltage Source3/RConn1
  Three-Phase Breaker1/LConn3 -- Three-Phase V-I Measurement1/RConn3
  Three-Phase V-I Measurement/RConn3 -- Inv_g_C/RConn1
  Inv_g_A/RConn1 -- Three-Phase V-I Measurement/RConn1
  Three-Phase V-I Measurement4/RConn1 -- Three-Phase V-I Measurement2/LConn1
  Three-Phase V-I Measurement4/RConn2 -- Three-Phase V-I Measurement2/LConn2
  Three-Phase V-I Measurement2/LConn3 -- Three-Phase V-I Measurement4/RConn3
  Controlled Voltage Source1/LConn1 -- Ground/LConn1
  Three-Phase Breaker1/LConn2 -- Three-Phase V-I Measurement1/RConn2
  Three-Phase Breaker1/LConn1 -- Three-Phase V-I Measurement1/RConn1
  Three-Phase V-I Measurement1/LConn1 -- L/RConn1
  Three-Phase V-I Measurement1/LConn2 -- L/RConn2
  Three-Phase V-I Measurement1/LConn3 -- L/RConn3
  Controlled Voltage Source/LConn1 -- Ground1/LConn1
  Controlled Voltage Source3/LConn1 -- Ground2/LConn1
  Three-Phase Breaker1/RConn1 -- Three-Phase V-I Measurement/LConn1
  Three-Phase V-I Measurement/LConn2 -- Three-Phase Breaker1/RConn2
  Three-Phase V-I Measurement/LConn3 -- Three-Phase Breaker1/RConn3
  L/LConn1 -- Three-Phase V-I Measurement2/RConn1
  L/LConn2 -- Three-Phase V-I Measurement2/RConn2
  L/LConn3 -- Three-Phase V-I Measurement2/RConn3

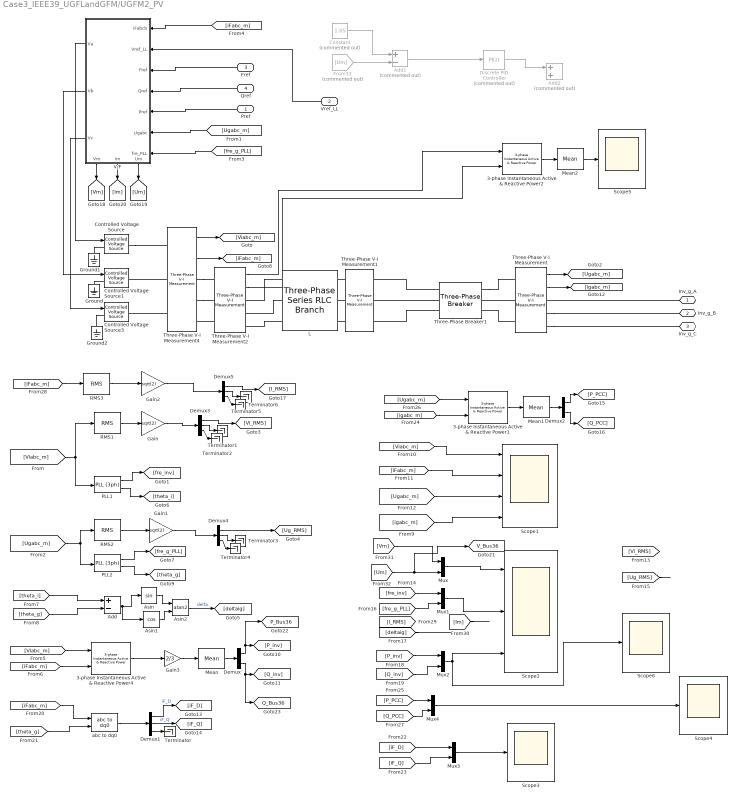
== system Case3_IEEE39_UGFLandGFM/UGFM2_PV ==
  Pref : Inport
  Vref_LL : Inport  Port=2
  Fref : Inport  Port=3
  Qref : Inport  Port=4
  3-phase Instantaneous Active & Reactive Power1 : powerlib_extras/Measurements/3-phase  Instantaneous  Active & Reactive Power
  3-phase Instantaneous Active & Reactive Power2 : powerlib_extras/Measurements/3-phase  Instantaneous  Active & Reactive Power
  3-phase Instantaneous Active & Reactive Power4 : powerlib_extras/Measurements/3-phase  Instantaneous  Active & Reactive Power
  Add : Sum  Inputs=+-
  Add1 : Sum  Commented=on  Inputs=+-
  Add2 : Sum  Commented=on
  Asin : Trigonometry
  Asin1 : Trigonometry  Operator=cos
  Asin2 : Trigonometry  Operator=atan2
  Constant : Constant  Commented=on  Value=1.05
  Controlled Voltage Source : spsControlledVoltageSourceLib/Controlled Voltage Source  Initialize=on  Source_Type=DC  Amplitude=300  Phase=0  Frequency=60  Measurements=None
  Controlled Voltage Source1 : spsControlledVoltageSourceLib/Controlled Voltage Source  Initialize=on  Source_Type=DC  Amplitude=300  Phase=-120  Frequency=60  Measurements=None
  Controlled Voltage Source3 : spsControlledVoltageSourceLib/Controlled Voltage Source  Initialize=on  Source_Type=DC  Amplitude=300  Phase=120  Frequency=60  Measurements=None
  Demux : Demux  Outputs=2
  Demux{1,3..5} (4 alike) : Demux  Outputs=3
  Demux2 : Demux  Outputs=2
  Discrete PID Controller : slpidlib/PID Controller  Commented=on  Controller=PI  Form=Parallel  TimeDomain=Discrete-time  UseExternalTs=off  SampleTime=-1  IntegratorMethod=Forward Euler  FilterMethod=Forward Euler  ControllerParametersSource=internal  P=1  I=50  UseKiTs=off  D=0  UseExternalDerivativeSource=off  N=100  UseFilter=on  TunerSelectOption=Transfer Function Based (PID Tuner App)  InitialConditionSource=internal  InitialConditionForIntegrator=0  InitialConditionForFilter=0  DifferentiatorICPrevScaledInput=0  ExternalReset=none  TrackingMode=off  Kt=1  LimitOutput=off  SatLimitsSource=internal  UpperSaturationLimit=inf  LowerSaturationLimit=-inf  LinearizeAsGain=off  AntiWindupMode=none  Kb=1  LimitIntegrator=off  UpperIntegratorSaturationLimit=inf  LowerIntegratorSaturationLimit=-inf  POutMin=[]  POutMax=[]  IOutMin=[]  IOutMax=[]  DOutMin=[]  DOutMax=[]  NOutMin=[]  NOutMax=[]  SumOutMin=[]  SumOutMax=[]  SaturationOutMin=[]  SaturationOutMax=[]  PParamMin=[]  PParamMax=[]  IParamMin=[]  IParamMax=[]  DParamMin=[]  DParamMax=[]  NParamMin=[]  NParamMax=[]  KbParamMin=[]  KbParamMax=[]  KtParamMin=[]  KtParamMax=[]  KbOutMin=[]  KbOutMax=[]  KtOutMin=[]  KtOutMax=[]  IntegratorOutMin=[]  IntegratorOutMax=[]  FilterOutMin=[]  FilterOutMax=[]  SumI1OutMin=[]  SumI1OutMax=[]  SumI2OutMin=[]  SumI2OutMax=[]  SumI3OutMin=[]  SumI3OutMax=[]  SumI4OutMin=[]  SumI4OutMax=[]  SumDOutMin=[]  SumDOutMax=[]  DifferentiatorOutMin=[]  DifferentiatorOutMax=[]  FilterDiffOutCoefMin=[]  FilterDiffOutCoefMax=[]  ReciprocalOutMin=[]  ReciprocalOutMax=[]  SumDenOutMin=[]  SumDenOutMax=[]  SumNumOutMin=[]  SumNumOutMax=[]  DivideOutMin=[]  DivideOutMax=[]  UdiffTsProdOutMin=[]  UdiffTsProdOutMax=[]  NTsProdOutMin=[]  NTsProdOutMax=[]  UintegralTsProdOutMin=[]  UintegralTsProdOutMax=[]  UngainTsProdOutMin=[]  UngainTsProdOutMax=[]  ClampingZeroOutDataTypeStr=Inherit: Inherit via back propagation  ClampingZeroOutMin=[]  ClampingZeroOutMax=[]  FilterDenConstantOutDataTypeStr=Inherit: Inherit via back propagation  FilterDenConstantOutMin=[]  FilterDenConstantOutMax=[]  PCopyOutDataTypeStr=Inherit: Inherit via back propagation  PCopyOutMin=[]  PCopyOutMax=[]  NCopyOutDataTypeStr=Inherit: Inherit via back propagation  NCopyOutMin=[]  NCopyOutMax=[]  IntegratorContinuousStateAttributes=''  IntegratorStateMustResolveToSignalObject=off  IntegratorRTWStateStorageClass=Auto  FilterContinuousStateAttributes=''  FilterStateMustResolveToSignalObject=off  FilterRTWStateStorageClass=Auto  ParallelPVariant=InternalParameters  IdealPVariant=Disabled  IVariant=InternalParameters  DVariant=Disabled  IntegratorVariant=Discrete  SatVariant=Disabled  AWVariant=Passthrough  PCopyVariant=Disabled  TRVariant=Disabled  FdbkBlocksVariant=Forward  IdealPFdbkVariant=Disabled  SatFdbkVariant=Disabled  DerivativeFilterVariant=Disabled  NVariant=Disabled  NCopyVariant=Disabled_SignalSpec  FilterICVariant=Disabled  IntegratorICVariant=InternalICs  ExternalResetVariant=Disabled  TRSumVariant=Passthrough  SumFdbkVariant=Disabled  SumVariant=Sum_PI  TsampFilterVariant=InternalTs  TsampNgainVariant=Passthrough  TsampIntegralVariant=Disabled_SignalSpec  ExternalSaturationOutDataTypeStr=Inherit: Same as second input  DerivativeSourceVariant=Disabled
      settings: LibrarySourceBlock=simulink/Discrete/Discrete PID Controller
  From33 : From  Commented=on  GotoTag=Um
  Gain : Gain  Gain=sqrt(2)
  Gain1 : Gain  Gain=sqrt(2)
  Gain2 : Gain  Gain=sqrt(2)
  Gain3 : Gain  Gain=2/3
  Ground : spsGroundLib/Ground  LConnTagsString=a
  Ground1 : spsGroundLib/Ground  LConnTagsString=a
  Ground2 : spsGroundLib/Ground  LConnTagsString=a
  L : spsThreePhaseSeriesRLCBranchLib/Three-Phase Series RLC Branch  LConnTagsString=A|B|C  RConnTagsString=A|B|C  BranchType=RL  Resistance=0.01*Vbase^2/Sbase  Inductance=0.05*(Vbase^2/Sbase/377)  Capacitance=1.0  Measurements=None
  Mean : spsMeanLib/Mean  Freq=60  Vinit=0  Ts=5e-4
  Mean1 : spsMeanLib/Mean  Freq=60  Vinit=0  Ts=1e-4
  Mean2 : spsMeanLib/Mean  Freq=60  Vinit=0  Ts=5e-4
  Mux{,1..4} (5 alike) : Mux  Inputs=2
  PLL1 : spsPLL3phLib/PLL (3ph)  Fmin=35  Par_Init=[0, 60]  ParK=[180, 3200, 1]  TcD=1e-4  MaxRateChangeFreq=12  FilterCutOffFreq=25  Ts=1e-5  AGC=on
  PLL2 : spsPLL3phLib/PLL (3ph)  Fmin=35  Par_Init=[0, 60]  ParK=[180, 3200, 1]  TcD=1e-4  MaxRateChangeFreq=12  FilterCutOffFreq=25  Ts=1e-5  AGC=on
  RMS1 : spsRMSLib/RMS  TrueRMS=on  Freq=60  RMSInit=1  Ts=1e-4
  RMS2 : spsRMSLib/RMS  TrueRMS=on  Freq=60  RMSInit=1  Ts=1e-4
  RMS3 : spsRMSLib/RMS  TrueRMS=on  Freq=60  RMSInit=1  Ts=5e-4
  Scope1 : Scope  NumInputPorts=4
  Scope2 : Scope  NumInputPorts=3
  Scope{3..6} (4 alike) : Scope
  Terminator{,1..6} (7 alike) : Terminator
  Three-Phase V-I Measurement : spsThreePhaseVIMeasurementLib/Three-Phase V-I Measurement  VoltageMeasurement=phase-to-ground  SetLabelV=off  LabelV=Vabc  Vpu=on  VpuLL=off  CurrentMeasurement=yes  SetLabelI=off  LabelI=Iabc  Ipu=on  Pbase=Sbase  Vbase=Vbase  OutputType=Complex  PhasorSimulation=off  PSBequivalent=0
  Three-Phase V-I Measurement1 : spsThreePhaseVIMeasurementLib/Three-Phase V-I Measurement  VoltageMeasurement=no  SetLabelV=off  LabelV=Vabc  Vpu=off  VpuLL=off  CurrentMeasurement=no  SetLabelI=off  LabelI=Iabc  Ipu=off  Pbase=1e5  Vbase=380  OutputType=Complex  PhasorSimulation=off  PSBequivalent=0
  Three-Phase V-I Measurement2 : spsThreePhaseVIMeasurementLib/Three-Phase V-I Measurement  VoltageMeasurement=phase-to-ground  SetLabelV=off  LabelV=Vabc  Vpu=off  VpuLL=off  CurrentMeasurement=yes  SetLabelI=off  LabelI=Iabc  Ipu=off  Pbase=Sbase  Vbase=Vbase  OutputType=Complex  PhasorSimulation=off  PSBequivalent=0
  Three-Phase V-I Measurement4 : spsThreePhaseVIMeasurementLib/Three-Phase V-I Measurement  VoltageMeasurement=phase-to-ground  SetLabelV=off  LabelV=u  Vpu=on  VpuLL=off  CurrentMeasurement=yes  SetLabelI=off  LabelI=iFabcp3  Ipu=on  Pbase=Sbase  Vbase=Vbase  OutputType=Complex  PhasorSimulation=off  PSBequivalent=0
  Three-Phase Breaker1 : spsThreePhaseBreakerLib/Three-Phase Breaker  InitialState=open  SwitchA=on  SwitchB=on  SwitchC=on  SwitchTimes=[0.1]  External=off  BreakerResistance=0.0001  SnubberResistance=1e8  SnubberCapacitance=inf  Measurements=None
  V/F : Subsystem
      settings: PortSchema="{\"entries\":[{\"content\":{\"sides\":[{\"content\":{\"connectorIds\":[\"In1\",\"In2\",\"In3\",\"In4\",\"In5\",\"In6\",\"In7\"]},\"type\":\"ConnectorPlacement.EquallySpacedRectSide\",\"uuid\":\"ccc7dc11-36db-4369-953c-0655fd1e2442\"},{\"content\":{\"connectorIds\":[\"Out1\",\"Out2\",\"Out3\"],\"side\":\"RIGHT\"},\"type\":\"ConnectorPlacement.EquallySpacedRectSide\",\"uuid\":\"5735cf9b-d8e4-4bce-b2db-12738d0d9e4d\"},{\"content\":{\"side\":\"TOP\"},\"type\":\"ConnectorPlacement.EquallySpacedRectSide\",\"uuid\":\"e010782d-2644-4ebf-978f-8395ad947d0e\"},{\"content\":{\"connectorIds\":[\"Out4\",\"Out5\",\"Out6\"],\"side\":\"BOTTOM\"},\"type\":\"ConnectorPlacement.EquallySpacedRectSide\",\"uuid\":\"5965ef6f-6121-4d63-9a5a-1f7a3d153058\"}]},\"type\":\"ConnectorPlacement.EquallySpacedConnector\",\"uuid\":\"be33ea6e-20ef-4fc3-81eb-341d11cc9c18\"}],\"packageUris\":[\"http://schema.mathworks.com/mf0/Connector/R2020b\"],\"version\":\"1.0\"}"
  abc to dq0 : spsabctodq0Lib/abc to dq0  Alignment=90 degrees behind phase A axis
  Inv_g_A : PMIOPort  Side=Right
  Inv_g_B : PMIOPort  Port=2  Side=Right
  Inv_g_C : PMIOPort  Port=3  Side=Right
  tag scope: P_Bus36=global, Q_Bus36=global, V_Bus36=global
  wires:
  Three-Phase V-I Measurement/1 -> [Ugabc_m]
  V/F/2(Vb) -> Controlled Voltage Source1/1
  V/F/3(Vc) -> Controlled Voltage Source3/1
  Pref/1 -> V/F/5(Pref)
  Qref/1 -> V/F/4(Qref)
  Fref/1 -> V/F/3(Fref)
  RMS1/1 -> Gain/1
  Three-Phase V-I Measurement4/1 -> [Viabc_m]
  [Viabc_m] -> RMS1/1, PLL1/1
  PLL1/2 -> [theta_i]
  PLL1/1 -> [fre_inv]
  [Ugabc_m] -> V/F/6(Ugabc)
  [Ugabc_m] -> PLL2/1, RMS2/1
  RMS2/1 -> Gain1/1
  PLL2/2 -> [theta_g]
  PLL2/1 -> [fre_g_PLL]
  Three-Phase V-I Measurement4/2 -> [iFabc_m]
  [iFabc_m] -> V/F/1(iFabcb)
  [Viabc_m] -> 3-phase Instantaneous Active & Reactive Power4/1
  [iFabc_m] -> 3-phase Instantaneous Active & Reactive Power4/2
  Mean/1 -> Demux/1
  Demux/1 -> [P_Bus36], [P_inv]
  Demux/2 -> [Q_Bus36], [Q_inv]
  Three-Phase V-I Measurement/2 -> [igabc_m]
  [Viabc_m] -> Scope1/1
  [iFabc_m] -> Scope1/2
  [Ugabc_m] -> Scope1/3
  [igabc_m] -> Scope1/4
  [fre_inv] -> Mux1/1
  [Ug_RMS] -> ?
  Mux/1 -> Scope2/1
  [fre_g_PLL] -> Mux1/2
  Mux1/1 -> Scope2/2
  [deltaig] -> ?
  [P_inv] -> Mux2/1
  [Q_inv] -> Mux2/2
  Mux2/1 -> Scope2/3, Scope6/1
  Gain/1 -> Demux3/1
  [fre_g_PLL] -> V/F/7(fre_PLL)
  [theta_i] -> Add/1
  Add/1 -> Asin/1, Asin1/1
  [theta_g] -> Add/2
  Asin/1 -> Asin2/1
  Asin1/1 -> Asin2/2
  Asin2/1 -> [deltaig]  "delta"
  [iFabc_m] -> abc to dq0/1
  [theta_g] -> abc to dq0/2
  abc to dq0/1 -> Demux1/1
  Demux1/3 -> Terminator/1
  Demux1/1 -> [iF_D]  "iF_D"
  Demux1/2 -> [iF_Q]  "iF_Q"
  [iF_D] -> Mux3/1
  [iF_Q] -> Mux3/2
  Mux3/1 -> Scope3/1
  V/F/1(Va) -> Controlled Voltage Source/1
  Demux2/2 -> [Q_PCC]
  [Ugabc_m] -> 3-phase Instantaneous Active & Reactive Power1/1
  [igabc_m] -> 3-phase Instantaneous Active & Reactive Power1/2
  Mean1/1 -> Demux2/1
  Demux2/1 -> [P_PCC]
  3-phase Instantaneous Active & Reactive Power1/1 -> Mean1/1
  [P_PCC] -> Mux4/1
  [Q_PCC] -> Mux4/2
  Mux4/1 -> Scope4/1
  Demux3/1 -> [Vi_RMS]
  Demux3/2 -> Terminator1/1
  Demux3/3 -> Terminator2/1
  Demux4/3 -> Terminator4/1
  Demux4/1 -> [Ug_RMS]
  Demux4/2 -> Terminator3/1
  Gain1/1 -> Demux4/1
  [iFabc_m] -> RMS3/1
  RMS3/1 -> Gain2/1
  Demux5/3 -> Terminator6/1
  Demux5/1 -> [I_RMS]
  Demux5/2 -> Terminator5/1
  Gain2/1 -> Demux5/1
  Three-Phase V-I Measurement2/1 -> 3-phase Instantaneous Active & Reactive Power2/1
  Mean2/1 -> Scope5/1
  Three-Phase V-I Measurement2/2 -> 3-phase Instantaneous Active & Reactive Power2/2
  3-phase Instantaneous Active & Reactive Power2/1 -> Mean2/1
  Gain3/1 -> Mean/1
  3-phase Instantaneous Active & Reactive Power4/1 -> Gain3/1
  [Vm] -> Mux/1
  [Um] -> [V_Bus36], Mux/2
  [Im] -> ?
  V/F/5(Im) -> [Im]
  V/F/6(Vm) -> [Vm]
  V/F/4(Um) -> [Um]
  From33/1 -> Add1/2
  Constant/1 -> Add1/1
  Add1/1 -> Discrete PID Controller/1
  Discrete PID Controller/1 -> Add2/1
  Vref_LL/1 -> V/F/2(Vref_LL)
  connections:
  Three-Phase V-I Measurement/RConn2 -- Inv_g_B/RConn1
  Three-Phase V-I Measurement4/LConn2 -- Controlled Voltage Source1/RConn1
  Controlled Voltage Source/RConn1 -- Three-Phase V-I Measurement4/LConn1
  Three-Phase V-I Measurement4/LConn3 -- Controlled Voltage Source3/RConn1
  Three-Phase Breaker1/LConn3 -- Three-Phase V-I Measurement1/RConn3
  Three-Phase V-I Measurement/RConn3 -- Inv_g_C/RConn1
  Inv_g_A/RConn1 -- Three-Phase V-I Measurement/RConn1
  Three-Phase V-I Measurement4/RConn1 -- Three-Phase V-I Measurement2/LConn1
  Three-Phase V-I Measurement4/RConn2 -- Three-Phase V-I Measurement2/LConn2
  Three-Phase V-I Measurement2/LConn3 -- Three-Phase V-I Measurement4/RConn3
  Controlled Voltage Source1/LConn1 -- Ground/LConn1
  Three-Phase Breaker1/LConn2 -- Three-Phase V-I Measurement1/RConn2
  Three-Phase Breaker1/LConn1 -- Three-Phase V-I Measurement1/RConn1
  Three-Phase V-I Measurement1/LConn1 -- L/RConn1
  Three-Phase V-I Measurement1/LConn2 -- L/RConn2
  Three-Phase V-I Measurement1/LConn3 -- L/RConn3
  Controlled Voltage Source/LConn1 -- Ground1/LConn1
  Controlled Voltage Source3/LConn1 -- Ground2/LConn1
  Three-Phase Breaker1/RConn1 -- Three-Phase V-I Measurement/LConn1
  Three-Phase V-I Measurement/LConn2 -- Three-Phase Breaker1/RConn2
  Three-Phase V-I Measurement/LConn3 -- Three-Phase Breaker1/RConn3
  L/LConn1 -- Three-Phase V-I Measurement2/RConn1
  L/LConn2 -- Three-Phase V-I Measurement2/RConn2
  L/LConn3 -- Three-Phase V-I Measurement2/RConn3
